simulink model "series_series"  (R2020b)
settings: Solver=VariableStepAuto  StartTime=0.0  StopTime=5e-3  RelTol=1e-3
values from neighbouring files (symbols this model uses):
  Cs = 1/(wo^2*Ls)    (= 5.11723149709e-08)    [deneme_tahtasi_error.m]    (also in parallel_series_errorpercentage.m; parallel_series_simulationout.m; series_series_errorpercentage_x.m; series_series_simulationout.m = 1.65557489612e-08)
  deltaM = i    [parallel_series_simulationout.m]    (also in series_series_simulationout.m)
  fop = f_i    [parallel_series_simulationout.m]    (also in series_series_simulationout.m)
  Ls = 22e-6    (= 2.2e-05)    [deneme_tahtasi_error.m]    (also in parallel_series_errorpercentage.m; parallel_series_simulationout.m; series_series_errorpercentage_x.m; series_series_simulationout.m = 6.8e-05)
libraries: powerlib x19, powerlib_meascontrol x2
settings Model: Creator=oguna  LastModifiedBy=oguna

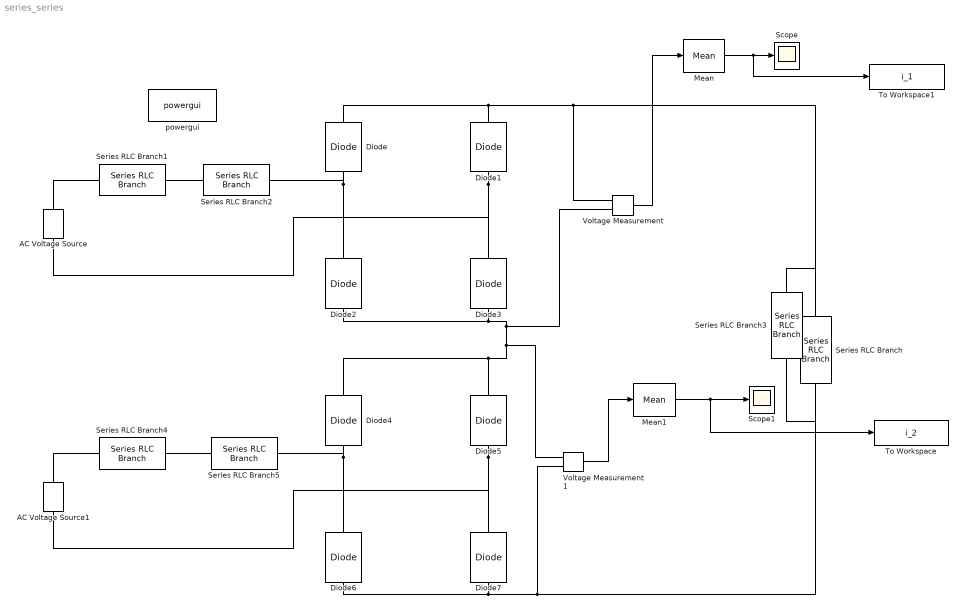
== system series_series ==
  AC Voltage Source : powerlib/Electrical Sources/AC Voltage Source  Amplitude=100  Phase=0  Frequency=fop  SampleTime=0  Measurements=None  BusType=swing  Pref=10e3  Qref=0  Qmin=-inf  Qmax=+inf
  AC Voltage Source1 : powerlib/Electrical Sources/AC Voltage Source  Amplitude=100*(1-deltaM)  Phase=0  Frequency=fop  SampleTime=0  Measurements=None  BusType=swing  Pref=10e3  Qref=0  Qmin=-inf  Qmax=+inf
  Diode{,1..7} (8 alike) : powerlib/Power Electronics/Diode  Ron=0  Lon=0  Vf=0  IC=0  UseSnubber=0  Rs=inf  Cs=0  Measurements=off
  Mean : powerlib_meascontrol/Measurements/Mean  Freq=fop  Vinit=0  Ts=0
  Mean1 : powerlib_meascontrol/Measurements/Mean  Freq=fop  Vinit=0  Ts=0
  Scope : Scope
  Scope1 : Scope
  Series RLC Branch : powerlib/Elements/Series RLC Branch  LConnTagsString=__new0  RConnTagsString=__new0  BranchType=R  Resistance=80  Inductance=1e-3  SetiL0=off  InitialCurrent=0  Capacitance=1e-6  Setx0=off  InitialVoltage=0  Measurements=None
  Series RLC Branch1 : powerlib/Elements/Series RLC Branch  LConnTagsString=__new0  RConnTagsString=__new0  BranchType=L  Resistance=13  Inductance=Ls  SetiL0=off  InitialCurrent=0  Capacitance=1e-6  Setx0=off  InitialVoltage=0  Measurements=None
  Series RLC Branch2 : powerlib/Elements/Series RLC Branch  LConnTagsString=__new0  RConnTagsString=__new0  BranchType=RC  Resistance=0.001  Inductance=1e-3  SetiL0=off  InitialCurrent=0  Capacitance=Cs  Setx0=off  InitialVoltage=0  Measurements=None
  Series RLC Branch3 : powerlib/Elements/Series RLC Branch  LConnTagsString=__new0  RConnTagsString=__new0  BranchType=RC  Resistance=0.0001  Inductance=1e-3  SetiL0=off  InitialCurrent=0  Capacitance=10e-6  Setx0=off  InitialVoltage=0  Measurements=None
  Series RLC Branch4 : powerlib/Elements/Series RLC Branch  LConnTagsString=__new0  RConnTagsString=__new0  BranchType=L  Resistance=13  Inductance=Ls  SetiL0=off  InitialCurrent=0  Capacitance=1e-6  Setx0=off  InitialVoltage=0  Measurements=None
  Series RLC Branch5 : powerlib/Elements/Series RLC Branch  LConnTagsString=__new0  RConnTagsString=__new0  BranchType=RC  Resistance=0.001  Inductance=1e-3  SetiL0=off  InitialCurrent=0  Capacitance=Cs  Setx0=off  InitialVoltage=0  Measurements=None
  To Workspace : ToWorkspace  VariableName=i_2  SampleTime=-1
      settings: MaxDataPoints=15  Decimation=3
  To Workspace1 : ToWorkspace  VariableName=i_1  SampleTime=-1
      settings: MaxDataPoints=15  Decimation=3
  Voltage Measurement : powerlib/Measurements/Voltage Measurement  PhasorSimulation=off  OutputType=Complex  PSBequivalent=0
  Voltage Measurement1 : powerlib/Measurements/Voltage Measurement  PhasorSimulation=off  OutputType=Complex  PSBequivalent=0
  powergui : powerlib/powergui  Priority=1  SimulationMode=Continuous  SampleTime=50e-6  frequency=60  Iterations=50  frequencyindice=200000  Pbase=100e6  ErrMax=1e-4  UnitsV=kV  UnitsW=MW  buscounter=0  FunctionMessages=off  echomessages=off  EnableUseOfTLC=off  CurrentSourceSwitches=off  DisableSnubberDevices=off  DisableRonSwitches=off  DisableVfSwitches=off  DisplayEquations=off  AutomaticDiscreteSolvers=off  SolverType=Tustin/Backward Euler (TBE)  Interpol=off  ExternalGateDelay=off  methode=off  Ts=100  x0status=blocks  SPID=on  SwTol=0  HookPort=off  NonlinearTolerance=1e-4  nMaxIteration=100  ContinueOnMaxIteration=off  RestoreLinks=warning  ResistiveCurrentMeasurement=off  Frange=[0:2:500]  Ylog=off  Xlog=on  ShowGrid=off  save=off  variable=ZData  structure=0  ZoomFFT=off  StartTime=0.0  cycles=1  DisplayStyle=1  fundamental=60  FreqAxis=off  MaxFrequency=1000  frequencyindicesteady=1  RmsSteady=1  display=off
  wires:
  Voltage Measurement/1 -> Mean/1
  Voltage Measurement1/1 -> Mean1/1
  Mean1/1 -> To Workspace/1, Scope1/1
  Mean/1 -> To Workspace1/1, Scope/1
  connections:
  Diode7/LConn1 -- Series RLC Branch3/RConn1 -- Series RLC Branch/RConn1 -- Voltage Measurement1/LConn2 -- Diode6/LConn1
  Diode5/LConn1 -- AC Voltage Source1/LConn1 -- Diode7/RConn1
  Diode1/LConn1 -- AC Voltage Source/LConn1 -- Diode3/RConn1
  Diode1/RConn1 -- Series RLC Branch3/LConn1 -- Series RLC Branch/LConn1 -- Voltage Measurement/LConn1 -- Diode/RConn1
  AC Voltage Source/RConn1 -- Series RLC Branch1/RConn1
  AC Voltage Source1/RConn1 -- Series RLC Branch4/RConn1
  Diode4/LConn1 -- Diode6/RConn1 -- Series RLC Branch5/RConn1
  Series RLC Branch2/LConn1 -- Series RLC Branch1/LConn1
  Diode5/RConn1 -- Voltage Measurement1/LConn1 -- Voltage Measurement/LConn2 -- Diode3/LConn1 -- Diode2/LConn1 -- Diode4/RConn1
  Diode/LConn1 -- Series RLC Branch2/RConn1 -- Diode2/RConn1
  Series RLC Branch5/LConn1 -- Series RLC Branch4/LConn1
